simulink model "Ship_Control_Loop_H_Infinity_Standard_Saturation"  (R2024a)
settings: Solver=VariableStepAuto  StartTime=0.0  StopTime=150  RelTol=1e-3
values from neighbouring files (symbols this model uses):
  Heading_Variance_Noise = 0.5*(pi/180)    (= 0.00872664625997)    [Controller_Stochastic_Optimization.m]    (also in Cost_Function_Optimal_Tuning_Controller.m = -0.00872664625997; Frequency_Responses.m)
  Input_Matrix_Controller_Nominal = Input_Matrix_Controller_After_Reduction    [Aposteriori_Corrector_Order_Reduction.m]
  Input_Matrix_Nominal_Global = [Input_Matrix_Nominal Perturbation_Input_Matrix_Nominal]    [Controller_Stochastic_Optimization.m]    (also in Standard_H_Infinity_Controller_Tuning.m)
  Input_Measurement_Matrix_Controller_Nominal = Input_Measurement_Matrix_Controller_After_Reduction    [Aposteriori_Corrector_Order_Reduction.m]
  Input_Measurement_Matrix_Global_Nominal = [0 0]    [Controller_Stochastic_Optimization.m]    (also in Standard_H_Infinity_Controller_Tuning.m)
  Measurement_Matrix_Controller_Nominal = Measurement_Matrix_Controller_After_Reduction    [Aposteriori_Corrector_Order_Reduction.m]
  Measurement_Matrix_Ship_Wave_Nominal = [0 1 1 0]    [Controller_Stochastic_Optimization.m]    (also in Standard_H_Infinity_Controller_Tuning.m)
  Perturbation_Step = 1*(pi/180)    (= 0.0174532925199)    [Controller_Stochastic_Optimization.m]    (also in Cost_Function_Optimal_Tuning_Controller.m; Frequency_Responses.m)
  State_Matrix_Controller_Nominal = State_Matrix_Controller_After_Reduction    [Aposteriori_Corrector_Order_Reduction.m]
  State_Matrix_Ship_Wave_Nominal = [0 1 0 0 ... (first row only)    [Controller_Stochastic_Optimization.m]    (also in Standard_H_Infinity_Controller_Tuning.m)
  Step_Heading_Aimed = 30*(pi/180)    (= 0.523598775598)    [Controller_Stochastic_Optimization.m]    (also in Cost_Function_Optimal_Tuning_Controller.m; Frequency_Responses.m)
settings Model: Creator=gerar  LastModifiedBy=gerar

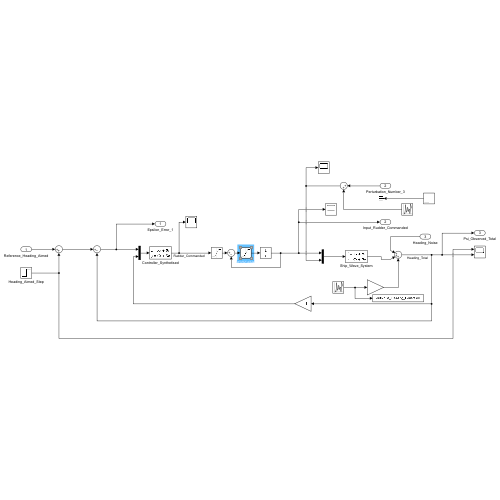
[thumbnail: Simulink's stored preview of the top-level diagram]
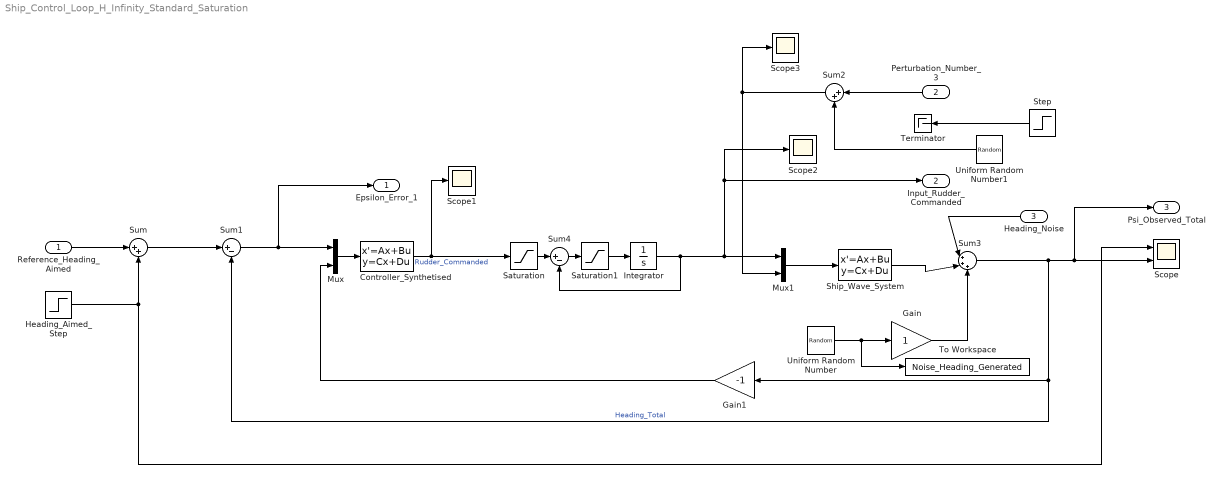
== system Ship_Control_Loop_H_Infinity_Standard_Saturation ==
  Reference_Heading_Aimed : Inport
  Perturbation_Number_3 : Inport  Port=2
  Heading_Noise : Inport  Port=3
  Controller_Synthetised : StateSpace  A=State_Matrix_Controller_Nominal  B=Input_Matrix_Controller_Nominal  C=Measurement_Matrix_Controller_Nominal  D=Input_Measurement_Matrix_Controller_Nominal  InitialCondition=0
  Gain : Gain  SaturateOnIntegerOverflow=on  OutDataTypeStr=Inherit: Same as input  ParamDataTypeStr=Inherit: Same as input
  Gain1 : Gain  Gain=-1  SaturateOnIntegerOverflow=on  OutDataTypeStr=Inherit: Same as input  ParamDataTypeStr=Inherit: Same as input
  Heading_Aimed_Step : Step  After=Step_Heading_Aimed  SampleTime=0
  Integrator : Integrator
  Mux : Mux  Inputs=2
  Mux1 : Mux  Inputs=2
  Saturation : Saturate  UpperLimit=35*(pi/180)  LowerLimit=-35*(pi/180)
  Saturation1 : Saturate  UpperLimit=5*(pi/180)  LowerLimit=-5*(pi/180)
  Scope : Scope  NumInputPorts=2
  Scope1 : Scope
  Scope2 : Scope
  Scope3 : Scope
  Ship_Wave_System : StateSpace  A=State_Matrix_Ship_Wave_Nominal  B=Input_Matrix_Nominal_Global  C=Measurement_Matrix_Ship_Wave_Nominal  D=Input_Measurement_Matrix_Global_Nominal  InitialCondition=0
  Step : Step  After=Perturbation_Step  SampleTime=0
  Sum : Sum  Inputs=|++
  Sum1 : Sum  Inputs=|+-
  Sum2 : Sum  Inputs=|++
  Sum3 : Sum  Inputs=|+++
  Sum4 : Sum  Inputs=|+-
  Terminator : Terminator
  To Workspace : ToWorkspace  VariableName=Noise_Heading_Generated  SaveFormat=Timeseries  SampleTime=-1
  Uniform Random Number : UniformRandomNumber  Minimum=-Heading_Variance_Noise  Maximum=Heading_Variance_Noise  SampleTime=1e-2
  Uniform Random Number1 : UniformRandomNumber  Minimum=-10*(pi/180)  Maximum=10*(pi/180)  SampleTime=1e-2
  Epsilon_Error_1 : Outport
  Input_Rudder_Commanded : Outport  Port=2
  Psi_Observed_Total : Outport  Port=3
  wires:
  Heading_Aimed_Step/1 -> Scope/1, Sum/2
  Reference_Heading_Aimed/1 -> Sum/1
  Sum/1 -> Sum1/1
  Sum1/1 -> Epsilon_Error_1/1, Mux/1
  Mux/1 -> Controller_Synthetised/1
  Controller_Synthetised/1 -> Saturation/1, Scope1/1  "Rudder_Commanded"
  Perturbation_Number_3/1 -> Sum2/1
  Sum2/1 -> Scope3/1, Mux1/2
  Mux1/1 -> Ship_Wave_System/1
  Ship_Wave_System/1 -> Sum3/2
  Heading_Noise/1 -> Sum3/1
  Uniform Random Number/1 -> To Workspace/1, Gain/1
  Gain/1 -> Sum3/3
  Sum3/1 -> Gain1/1, Sum1/2, Psi_Observed_Total/1, Scope/2  "Heading_Total"
  Gain1/1 -> Mux/2
  Saturation1/1 -> Integrator/1
  Integrator/1 -> Sum4/2, Scope2/1, Input_Rudder_Commanded/1, Mux1/1
  Saturation/1 -> Sum4/1
  Sum4/1 -> Saturation1/1
  Uniform Random Number1/1 -> Sum2/2
  Step/1 -> Terminator/1
